simulink model "dpll"  (Simulink 6.6)
settings: Solver=VariableStepDiscrete  StartTime=0.0  StopTime=50e-6  RelTol=1e-3
PostLoadFcn:
  | C2 = 17e-12;
  | C1 = 82e-12;
  | R1 = 23e3;
  | 
  | b = [0   1.000000000000000  -0.994711805058698];
  | a = [1.000000000000000  -1.969594171908450   0.969594171908450];
  | 
  | Ts = 1e-8;
undefined symbols (not defined in the file or in its folder): dfilt
libraries: dsparch4 x1, dspsigops x1, dspsnks4 x1
settings Model: Creator=Edwin Pasterkamp  LastModifiedBy=epasterk
settings DebuggingCC: AlgebraicLoopMsg=error  SignalResolutionControl=TryResolveAllWithWarning

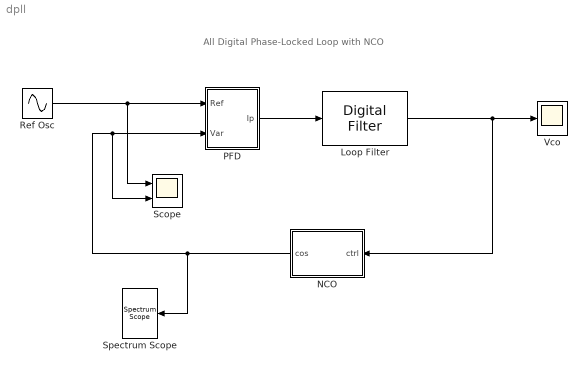
== system dpll ==
  note: All Digital Phase-Locked Loop with NCO
  Loop Filter : dsparch4/Digital Filter  DialogController=dspdialog.DigitalFilter  DialogControllerArgs=DataTag0  TypePopup=IIR (poles & zeros)  IIRFiltStruct=Direct form II transposed  AllPoleFiltStruct=Direct form  FIRFiltStruct=Direct form  CoeffSource=Specify via dialog  NumCoeffs=b  DenCoeffs=a  BiQuadCoeffs=[1 0.3 0.4 1 0.1 0.2]  LatticeCoeffs=[0.2 0.4]  denIgnore=on  FiltPerSampPopup=One filter per frame  IC=0  ICnum=0  ICden=0  roundingMode=Nearest  overflowMode=off  ScaleValues=1  scaleValueFracLength=14  stageInFracLength=15  stageOutFracLength=15  FilterSource=Specify via dialog  dfiltObjectName=dfilt.dffir([1 2 1])
  NCO : Subsystem  Orientation=left
  PFD : Subsystem
  Ref Osc : Sin  Frequency=2*pi*1.1e6  SampleTime=Ts
      settings: AttributesFormatString=%<Frequency> (rad/s)
  Scope : Scope  NumInputPorts=2
      settings: TimeRange=5e-005  YMin=-1.5~-1.5  YMax=1.5~1.5
  Spectrum Scope : dspsnks4/Spectrum Scope  Orientation=left  DialogController=dspdialog.SpectrumScope  DialogControllerArgs=DataTag1  SystemSampleTime=-1  ScopeProperties=on  Domain=Frequency  HorizSpan=1  UseBuffer=on  BufferSize=1024  Overlap=512  inpFftLenInherit=off  FFTlength=128  numAvg=2  DisplayProperties=off  AxisGrid=on  Memory=off  FrameNumber=on  AxisLegend=off  AxisZoom=off  OpenScopeAtSimStart=on  OpenScopeImmediately=off  FigPos=[7 356 1020 205]  AxisProperties=off  XUnits=Hertz  XRange=[0...Fs/2]  InheritXIncr=on  XIncr=1.0  XLabel=Samples  XLimit=Auto  YUnits=dB  XMax=1  XMin=0  YLabel=Magnitude-squared, dB  LineProperties=off  wintypeSpecScope=Kaiser  RsSpecScope=50  betaSpecScope=5  winsampSpecScope=Periodic
      settings: YMin=-66.7500151230149  YMax=24.4293933483218
  Vco : Scope
      settings: YMin=-30  YMax=30
  wires:
  PFD/1(Ip) -> Loop Filter/1
  Ref Osc/1 -> Scope/1, PFD/1(Ref)
  NCO/1(cos) -> Spectrum Scope/1, Scope/2, PFD/2(Var)
  Loop Filter/1 -> Vco/1, NCO/1(ctrl)

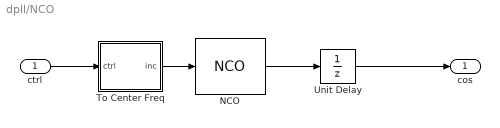
== system dpll/NCO ==
  ctrl : Inport
  NCO : dspsigops/NCO  DialogController=dspdialog.NCO  AccIncSrc=Input port  AccInc=16417  PhaseOffsetSrc=Specify via dialog  PhaseOffset=0  AccumWL=16  HasDither=off  DitherWL=5  PNgeneratorLength=12  HasPhaseQuantizer=off  TableDepth=14  HasOutputPhaseError=off  Formula=Cosine  DataType=double  OutputWL=16  OutputFL=14  CompMethod=Table lookup (no interpolation)  SampleTime=1/8000  SamplesPerFrame=1
  To Center Freq : Subsystem
  Unit Delay : UnitDelay  SampleTime=-1
  cos : Outport
  wires:
  To Center Freq/1(inc) -> NCO/1
  ctrl/1 -> To Center Freq/1(ctrl)
  NCO/1 -> Unit Delay/1
  Unit Delay/1 -> cos/1

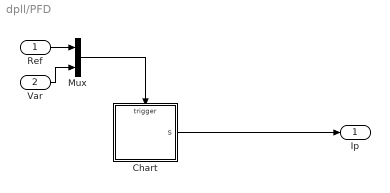
== system dpll/PFD ==
  Ref : Inport
  Var : Inport  Port=2
  Chart : Stateflow chart
  Mux : Mux  Inputs=2
  Ip : Outport
  wires:
  Chart/1(s) -> Ip/1
  Var/1 -> Mux/2
  Ref/1 -> Mux/1
  Mux/1 -> Chart/Trigger

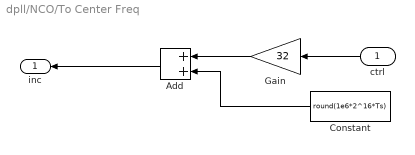
== system dpll/NCO/To Center Freq ==
  ctrl : Inport  Orientation=left
  Add : Sum  Orientation=left  OutScaling=2^-10  SampleTime=Ts  InputSameDT=on
  Constant : Constant  Orientation=left  Value=round(1e6*2^16*Ts)
  Gain : Gain  Orientation=left  Gain=32  OutDataTypeMode=Specify via dialog  OutDataType=sint(16)
  inc : Outport  Orientation=left
  wires:
  Constant/1 -> Add/2
  Add/1 -> inc/1
  Gain/1 -> Add/1
  ctrl/1 -> Gain/1

== stateflow chart PFD/Chart ==
  state Ahead
    s = -1;
  state InPhase
    s=0;
  state Behind
    s=1;
  Ahead -> InPhase : ref
  InPhase -> Behind [order 1] : ref
  InPhase -> Ahead [order 2] : var
  Behind -> InPhase : var
  (default) -> InPhase
  data: s output double
  events: ref input RISING_EDGE_EVENT; var input RISING_EDGE_EVENT
